simulink model "scenario_wind_integration"  (R2016b)
settings: Solver=ode23tb  StartTime=0.0  StopTime=2  RelTol=1e-3  EnableMultiTasking=on
undefined symbols (not defined in the file): sigbuilder_block
libraries: powerlib x28, powerlib_extras x7
settings Model: Creator=Amir  LastModifiedBy=Hosein
settings DataIOCC: LimitDataPoints=on  SaveFormat=Array  SignalLoggingSaveFormat=ModelDataLogs
settings OptimizationCC: ExpressionDepthLimit=2147483647  LifeSpan=inf
settings DebuggingCC: UnderspecifiedInitializationDetection=Classic  MergeDetectMultiDrivingBlocksExec=none  SolverPrmCheckMsg=warning  FcnCallInpInsideContextMsg=warning  StateNameClashWarn=warning  StrictBusMsg=Warning  SFUnexpectedBacktrackingDiag=warning  SFNoUnconditionalDefaultTransitionDiag=warning  SFExecutionAtInitializationDiag=none
settings HardwareCC: ProdBitPerPointer=32  ProdBitPerSizeT=32  ProdBitPerPtrDiffT=32  ProdLargestAtomicFloat=None  ProdIntDivRoundTo=Undefined  ProdEndianess=Unspecified  ProdWordSize=32  ProdHWDeviceType=32-bit Generic
settings ModelReferenceCC: PropagateSignalLabelsOutOfModel=off
settings GRTTargetCC: TargetLangStandard=C89/C90 (ANSI)  CombineOutputUpdateFcns=off  GRTInterface=on
settings ConfigComp: CovMetricSettings=dw  CovHtmlReporting=on  CovSaveCumulativeToWorkspaceVar=on  CovSaveSingleToWorkspaceVar=on  CovExternalEMLEnable=off

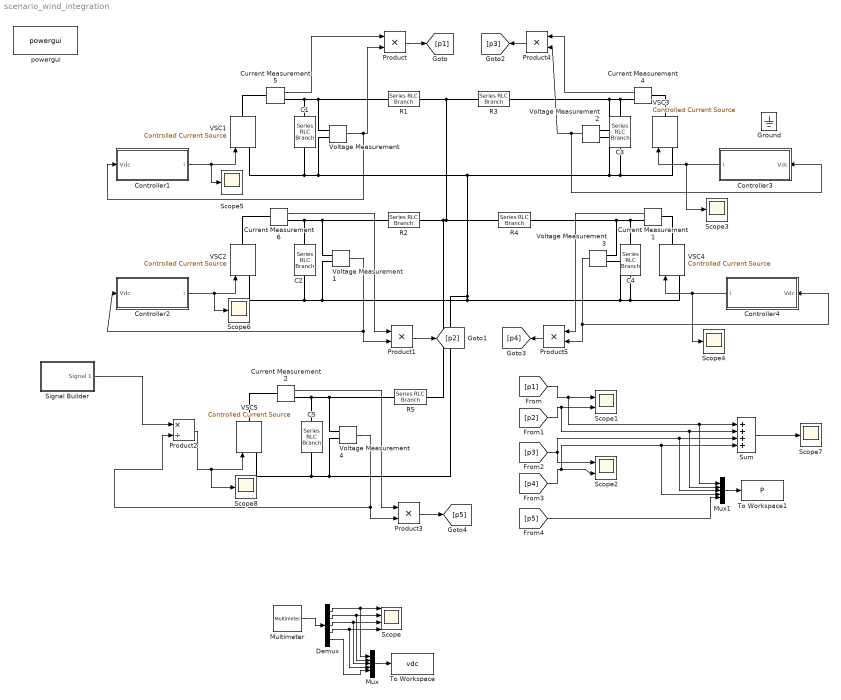
== system scenario_wind_integration ==
  C{1..5} (5 alike) : powerlib/Elements/Series RLC Branch  LConnTagsString=__new0  RConnTagsString=__new0  BranchType=C  Resistance=1  Inductance=1e-3  SetiL0=off  InitialCurrent=0  Capacitance=75e-6  Setx0=on  InitialVoltage=100e3  Measurements=Branch voltage
  Controller1 : Subsystem
  Controller2 : Subsystem
  Controller3 : Subsystem
  Controller4 : Subsystem
  Current Measurement{1..2,4..6} (5 alike) : powerlib/Measurements/Current Measurement  PhasorSimulation=off  OutputType=Complex  PSBequivalent=0
  Demux : Demux  Outputs=5
  Ground : powerlib/Elements/Ground  LConnTagsString=a
  Multimeter : powerlib/Measurements/Multimeter  PhasorSimulation=off  OutputType=Complex  sel=[1 2 3 4 5]  L=5  Gain=[1 1 1 1 1]  yselected={'Ub: C1','Ub: C2','Ub: C3','Ub: C4','Ub: C5'};  PSBOutputType=1  PSBequivalent=0  AxesSetting=[0,0.1,-100,100]  Display=0  SavedBlockNames=-11
  Mux : Mux  Inputs=5
  Mux1 : Mux  Inputs=5
  Product{,1,3..5} (5 alike) : Product  RndMeth=Zero
  Product2 : Product  Inputs=*/  RndMeth=Zero
  R1 : powerlib/Elements/Series RLC Branch  LConnTagsString=__new0  RConnTagsString=__new0  BranchType=R  Resistance=1.78  Inductance=141.5e-3  SetiL0=off  InitialCurrent=0  Capacitance=1e-6  Setx0=off  InitialVoltage=0  Measurements=None
  R2 : powerlib/Elements/Series RLC Branch  LConnTagsString=__new0  RConnTagsString=__new0  BranchType=R  Resistance=1.78  Inductance=141.5e-3  SetiL0=on  InitialCurrent=-1  Capacitance=1e-6  Setx0=off  InitialVoltage=0  Measurements=None
  R3 : powerlib/Elements/Series RLC Branch  LConnTagsString=__new0  RConnTagsString=__new0  BranchType=R  Resistance=1.78*0.5  Inductance=141.5e-3*0.5  SetiL0=on  InitialCurrent=0.5  Capacitance=1e-6  Setx0=off  InitialVoltage=0  Measurements=None
  R4 : powerlib/Elements/Series RLC Branch  LConnTagsString=__new0  RConnTagsString=__new0  BranchType=R  Resistance=1.78*0.75  Inductance=141.5e-3*0.75  SetiL0=on  InitialCurrent=0.5  Capacitance=1e-6  Setx0=off  InitialVoltage=0  Measurements=None
  R5 : powerlib/Elements/Series RLC Branch  LConnTagsString=__new0  RConnTagsString=__new0  BranchType=R  Resistance=1.78  Inductance=141.5e-3  SetiL0=on  InitialCurrent=-1  Capacitance=1e-6  Setx0=off  InitialVoltage=0  Measurements=None
  Scope : Scope  NumInputPorts=4
  Scope1 : Scope  NumInputPorts=2
  Scope2 : Scope  NumInputPorts=2
  Scope{3..8} (6 alike) : Scope
  Signal Builder : Subsystem  Tag=STV Subsys  LoadFcn=sigbuilder_block('load');  StartFcn=sigbuilder_block('start');  StopFcn=sigbuilder_block('stop');  ClipboardFcn=sigbuilder_block('clipboard');  mask(Sigbuilder block){tuvar=[0:10]}
      mask help: Sigbuilder GUI
      mask init:
      | if ~strcmp(get_param(bdroot(gcbh),'SimulationStatus'),'stopped') tuvar = sigbuilder_block('maskInit'); end
      settings: CopyFcn=sigbuilder_block('copy');  DeleteFcn=sigbuilder_block('delete');  ModelCloseFcn=sigbuilder_block('modelClose');  PreSaveFcn=sigbuilder_block('preSave');  PauseFcn=sigbuilder_block('pause')  ContinueFcn=sigbuilder_block('continue')  NameChangeFcn=sigbuilder_block('namechange');  OpenFcn=sigbuilder_block('open',[440.4 121.2 544.2 396 ]);  CloseFcn=sigbuilder_block('close');
      mask Display: plot(0,0,100,100,[10,10,40,40,10],[80,20,20,80,80],[40,10],[50,50], [40,27,10],[65,72,56],[40,25,25,10],[28,28,43,43]);
  Sum : Sum  Inputs=4
  To Workspace : ToWorkspace  VariableName=vdc  SampleTime=-1
  To Workspace1 : ToWorkspace  VariableName=P  SampleTime=-1
  VSC{1..5} (5 alike) : powerlib/Electrical Sources/Controlled Current Source  Initialize=on  Source_Type=AC  Amplitude=0  Phase=0  Frequency=0  Measurements=None
  Voltage Measurement{,1..4} (5 alike) : powerlib/Measurements/Voltage Measurement  PhasorSimulation=off  OutputType=Complex  PSBequivalent=0
  powergui : powerlib/powergui  Priority=1  SimulationMode=Discrete  SolverType=Tustin/Backward Euler (TBE)  SampleTime=1e-4  frequency=60  SPID=off  DisableSnubberDevices=off  DisableRonSwitches=off  DisableVfSwitches=off  SwTol=0  DisplayEquations=off  Interpol=off  ExternalGateDelay=off  methode=off  Ts=0  FunctionMessages=off  echomessages=off  HookPort=off  EnableUseOfTLC=off  x0status=blocks  frequencyindice=0  Pbase=100e6  ErrMax=1e-4  Iterations=50  UnitsV=kV  UnitsW=MW  buscounter=0  RestoreLinks=warning  ResistiveCurrentMeasurement=off  Frange=[0:2:500]  Ylog=off  Xlog=on  ShowGrid=off  save=off  variable=ZData  structure=0  ZoomFFT=on  StartTime=0.0  cycles=1  DisplayStyle=1  fundamental=60  FreqAxis=off  MaxFrequency=1000  frequencyindicesteady=1  RmsSteady=1  display=off
  wires:
  Controller4/1(i) -> VSC4/1, Scope4/1
  Controller3/1(i) -> VSC3/1, Scope3/1
  Controller1/1(i) -> VSC1/1, Scope5/1
  Controller2/1(i) -> VSC2/1, Scope6/1
  Multimeter/1 -> Demux/1
  Demux/1 -> Scope/1, Mux/1
  Demux/2 -> Scope/2, Mux/2
  Demux/3 -> Scope/3, Mux/3
  Demux/4 -> Scope/4, Mux/4
  Voltage Measurement/1 -> Product/2, Controller1/1(Vdc)
  Current Measurement6/1 -> Product1/1
  Voltage Measurement1/1 -> Product1/2, Controller2/1(Vdc)
  Product/1 -> [p1]
  Product1/1 -> [p2]
  [p1] -> Scope1/1, Sum/1, Mux1/1
  [p2] -> Scope1/2, Sum/2, Mux1/2
  Voltage Measurement2/1 -> Product4/2, Controller3/1(Vdc)
  Voltage Measurement3/1 -> Product5/2, Controller4/1(Vdc)
  Current Measurement4/1 -> Product4/1
  Current Measurement1/1 -> Product5/1
  Product4/1 -> [p3]
  Product5/1 -> [p4]
  [p3] -> Scope2/1, Sum/3, Mux1/3
  [p4] -> Scope2/2, Sum/4, Mux1/4
  Sum/1 -> Scope7/1
  Current Measurement5/1 -> Product/1
  Mux/1 -> To Workspace/1
  Signal Builder/1(Signal 1) -> Product2/1
  Mux1/1 -> To Workspace1/1
  Product2/1 -> VSC5/1, Scope8/1
  Current Measurement2/1 -> Product3/1
  Voltage Measurement4/1 -> Product3/2, Product2/2
  Product3/1 -> [p5]
  [p5] -> Mux1/5
  Demux/5 -> Mux/5
  connections:
  R1/LConn1 -- C1/LConn1 -- Current Measurement5/RConn1 -- Voltage Measurement/LConn1
  VSC1/LConn1 -- C1/RConn1 -- Voltage Measurement/LConn2 -- VSC3/LConn1 -- C3/RConn1 -- Voltage Measurement2/LConn2 -- VSC2/LConn1 -- C2/RConn1 -- Voltage Measurement1/LConn2 -- VSC4/LConn1 -- C4/RConn1 -- Voltage Measurement3/LConn2 -- Voltage Measurement4/LConn2 -- C5/RConn1 -- VSC5/LConn1
  R2/RConn1 -- R4/LConn1 -- R1/RConn1 -- R3/LConn1 -- R5/RConn1
  R3/RConn1 -- Voltage Measurement2/LConn1 -- C3/LConn1 -- Current Measurement4/RConn1
  R2/LConn1 -- C2/LConn1 -- Current Measurement6/RConn1 -- Voltage Measurement1/LConn1
  R4/RConn1 -- C4/LConn1 -- Current Measurement1/RConn1 -- Voltage Measurement3/LConn1
  Current Measurement5/LConn1 -- VSC1/RConn1
  Current Measurement6/LConn1 -- VSC2/RConn1
  Current Measurement1/LConn1 -- VSC4/RConn1
  Current Measurement4/LConn1 -- VSC3/RConn1
  R5/LConn1 -- Voltage Measurement4/LConn1 -- C5/LConn1 -- Current Measurement2/RConn1
  Current Measurement2/LConn1 -- VSC5/RConn1

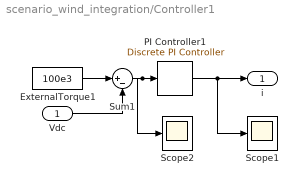
== system scenario_wind_integration/Controller1 ==
  Vdc : Inport
  ExternalTorque1 : Constant  Value=100e3
  PI Controller1 : powerlib_extras/Discrete  Control Blocks/Discrete PI Controller  Kp=10  Ki=10  Par_Limits=[0 -1000]  Init=0  Ts=1e-4
  Scope1 : Scope
  Scope2 : Scope
  Sum1 : Sum  Inputs=|+-
  i : Outport
  wires:
  ExternalTorque1/1 -> Sum1/1
  Vdc/1 -> Sum1/2
  Sum1/1 -> PI Controller1/1, Scope2/1
  PI Controller1/1 -> i/1, Scope1/1

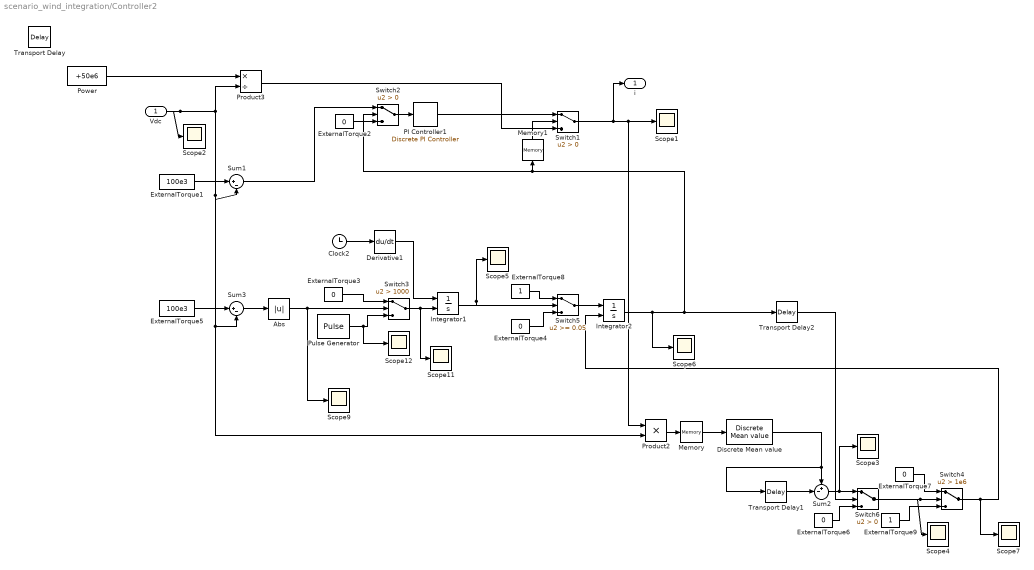
== system scenario_wind_integration/Controller2 ==
  Vdc : Inport
  Abs : Abs
  Clock2 : Clock
  Derivative1 : Derivative
  Discrete Mean value : powerlib_extras/Discrete Measurements/Discrete  Mean value  Freq=100  Vinit=0  Ts=1e-4
  ExternalTorque1 : Constant  Value=100e3
  ExternalTorque{2..4,6..7} (5 alike) : Constant  Value=0
  ExternalTorque5 : Constant  Value=100e3
  ExternalTorque8 : Constant
  ExternalTorque9 : Constant
  Integrator1 : Integrator  ExternalReset=either
  Integrator2 : Integrator  ExternalReset=either
  Memory : Memory
  Memory1 : Memory
  PI Controller1 : powerlib_extras/Discrete  Control Blocks/Discrete PI Controller  Kp=10  Ki=10  Par_Limits=[1000 -1000]  Init=0  Ts=1e-4
  Power : Constant  Value=+50e6
  Product2 : Product  Inputs=**  RndMeth=Zero
  Product3 : Product  Inputs=*/  RndMeth=Zero
  Pulse Generator : DiscretePulseGenerator  PulseType=Time based  Period=1e-4  PulseWidth=50
  Scope{1..7,9,11..12} (10 alike) : Scope
  Sum1 : Sum  Inputs=|+-
  Sum2 : Sum  Inputs=+-|
  Sum3 : Sum  Inputs=|+-
  Switch1 : Switch  Criteria=u2 > Threshold
  Switch2 : Switch  Criteria=u2 > Threshold
  Switch3 : Switch  Criteria=u2 > Threshold  Threshold=1000
  Switch4 : Switch  Criteria=u2 > Threshold  Threshold=1e6
  Switch5 : Switch  Threshold=0.05
  Switch6 : Switch  Criteria=u2 > Threshold
  Transport Delay : TransportDelay  DelayTime=0.05
  Transport Delay1 : TransportDelay  DelayTime=0.001
  Transport Delay2 : TransportDelay  DelayTime=0.1
  i : Outport
  wires:
  Sum1/1 -> Switch2/1
  ExternalTorque1/1 -> Sum1/1
  Power/1 -> Product3/1
  Product3/1 -> Switch1/3
  Switch2/1 -> PI Controller1/1
  PI Controller1/1 -> Switch1/1
  ExternalTorque2/1 -> Switch2/3
  Switch1/1 -> i/1, Scope1/1, Product2/1
  Switch3/1 -> Integrator1/2, Scope11/1
  Pulse Generator/1 -> Switch3/3, Scope12/1
  ExternalTorque3/1 -> Switch3/1
  Clock2/1 -> Derivative1/1
  Derivative1/1 -> Integrator1/1
  Abs/1 -> Switch3/2, Scope9/1
  Integrator1/1 -> Scope5/1, Switch5/2
  ExternalTorque4/1 -> Switch5/3
  Switch5/1 -> Integrator2/1
  ExternalTorque8/1 -> Switch5/1
  Integrator2/1 -> Scope6/1, Switch2/2, Memory1/1, Transport Delay2/1
  Vdc/1 -> Product3/2, Sum1/2, Product2/2, Sum3/2, Scope2/1
  Product2/1 -> Memory/1
  ExternalTorque9/1 -> Switch4/3
  ExternalTorque7/1 -> Switch4/1
  Discrete Mean value/1 -> Sum2/1, Transport Delay1/1
  Memory/1 -> Discrete Mean value/1
  Sum3/1 -> Abs/1
  ExternalTorque5/1 -> Sum3/1
  Memory1/1 -> Switch1/2
  Transport Delay1/1 -> Sum2/2
  Sum2/1 -> Switch6/1, Scope3/1
  Switch6/1 -> Switch4/2, Scope4/1
  ExternalTorque6/1 -> Switch6/3
  Switch4/1 -> Scope7/1, Integrator2/2
  Transport Delay2/1 -> Switch6/2

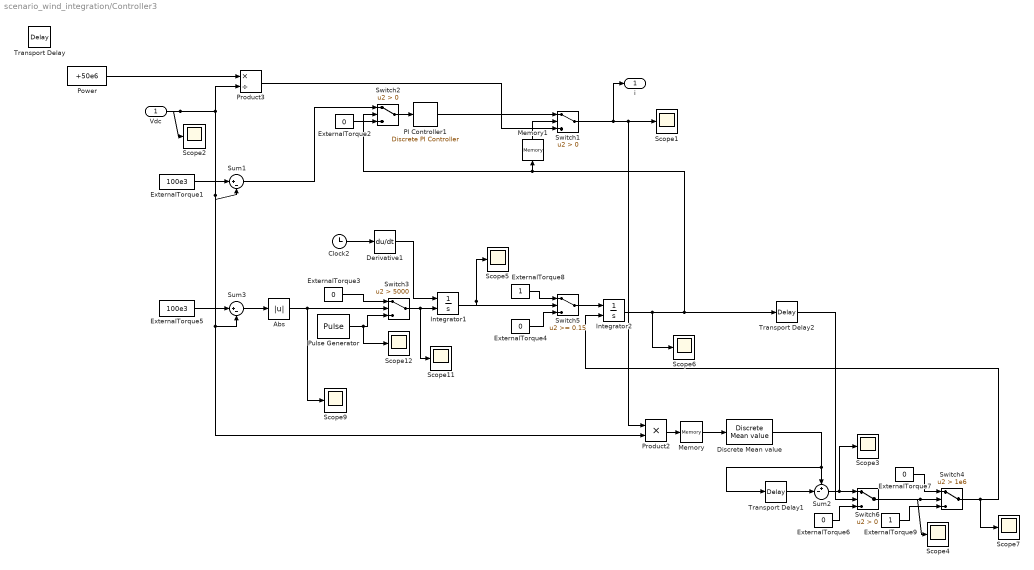
== system scenario_wind_integration/Controller3 ==
  Vdc : Inport
  Abs : Abs
  Clock2 : Clock
  Derivative1 : Derivative
  Discrete Mean value : powerlib_extras/Discrete Measurements/Discrete  Mean value  Freq=100  Vinit=0  Ts=1e-4
  ExternalTorque1 : Constant  Value=100e3
  ExternalTorque{2..4,6..7} (5 alike) : Constant  Value=0
  ExternalTorque5 : Constant  Value=100e3
  ExternalTorque8 : Constant
  ExternalTorque9 : Constant
  Integrator1 : Integrator  ExternalReset=either
  Integrator2 : Integrator  ExternalReset=either
  Memory : Memory
  Memory1 : Memory
  PI Controller1 : powerlib_extras/Discrete  Control Blocks/Discrete PI Controller  Kp=10  Ki=10  Par_Limits=[1000 -1000]  Init=0  Ts=1e-4
  Power : Constant  Value=+50e6
  Product2 : Product  Inputs=**  RndMeth=Zero
  Product3 : Product  Inputs=*/  RndMeth=Zero
  Pulse Generator : DiscretePulseGenerator  PulseType=Time based  Period=1e-4  PulseWidth=50
  Scope{1..7,9,11..12} (10 alike) : Scope
  Sum1 : Sum  Inputs=|+-
  Sum2 : Sum  Inputs=+-|
  Sum3 : Sum  Inputs=|+-
  Switch1 : Switch  Criteria=u2 > Threshold
  Switch2 : Switch  Criteria=u2 > Threshold
  Switch3 : Switch  Criteria=u2 > Threshold  Threshold=5000
  Switch4 : Switch  Criteria=u2 > Threshold  Threshold=1e6
  Switch5 : Switch  Threshold=0.15
  Switch6 : Switch  Criteria=u2 > Threshold
  Transport Delay : TransportDelay  DelayTime=0.05
  Transport Delay1 : TransportDelay  DelayTime=0.001
  Transport Delay2 : TransportDelay  DelayTime=0.1
  i : Outport
  wires:
  Transport Delay2/1 -> Switch6/2
  Switch4/1 -> Integrator2/2, Scope7/1
  ExternalTorque6/1 -> Switch6/3
  Switch6/1 -> Scope4/1, Switch4/2
  Sum2/1 -> Scope3/1, Switch6/1
  Transport Delay1/1 -> Sum2/2
  Memory1/1 -> Switch1/2
  ExternalTorque5/1 -> Sum3/1
  Sum3/1 -> Abs/1
  Memory/1 -> Discrete Mean value/1
  Discrete Mean value/1 -> Transport Delay1/1, Sum2/1
  ExternalTorque7/1 -> Switch4/1
  ExternalTorque9/1 -> Switch4/3
  Product2/1 -> Memory/1
  Vdc/1 -> Scope2/1, Sum3/2, Product2/2, Sum1/2, Product3/2
  Integrator2/1 -> Transport Delay2/1, Memory1/1, Switch2/2, Scope6/1
  ExternalTorque8/1 -> Switch5/1
  Switch5/1 -> Integrator2/1
  ExternalTorque4/1 -> Switch5/3
  Integrator1/1 -> Switch5/2, Scope5/1
  Abs/1 -> Scope9/1, Switch3/2
  Derivative1/1 -> Integrator1/1
  Clock2/1 -> Derivative1/1
  ExternalTorque3/1 -> Switch3/1
  Pulse Generator/1 -> Scope12/1, Switch3/3
  Switch3/1 -> Scope11/1, Integrator1/2
  Switch1/1 -> Product2/1, Scope1/1, i/1
  ExternalTorque2/1 -> Switch2/3
  PI Controller1/1 -> Switch1/1
  Switch2/1 -> PI Controller1/1
  Product3/1 -> Switch1/3
  Power/1 -> Product3/1
  ExternalTorque1/1 -> Sum1/1
  Sum1/1 -> Switch2/1

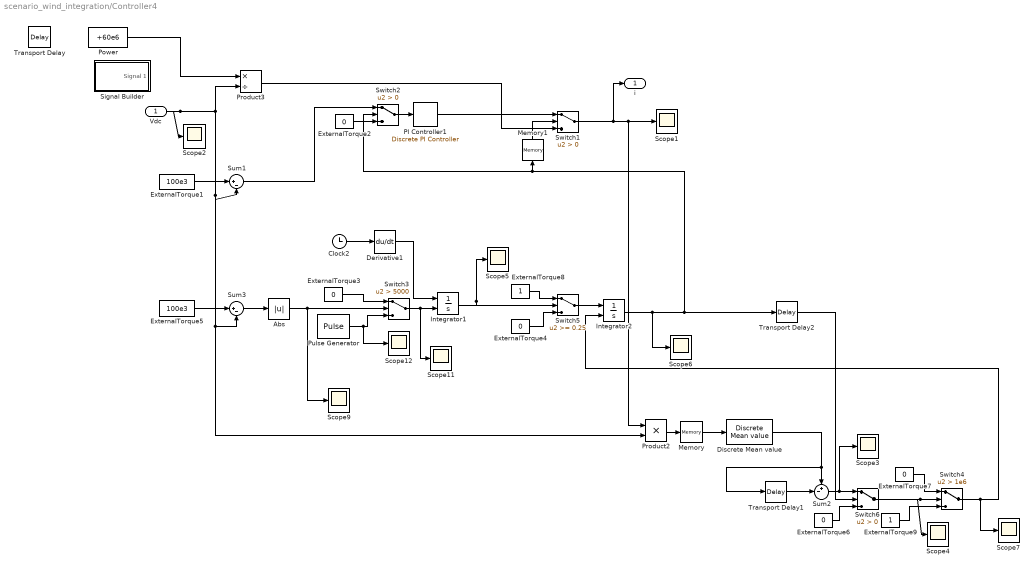
== system scenario_wind_integration/Controller4 ==
  Vdc : Inport
  Abs : Abs
  Clock2 : Clock
  Derivative1 : Derivative
  Discrete Mean value : powerlib_extras/Discrete Measurements/Discrete  Mean value  Freq=100  Vinit=0  Ts=1e-4
  ExternalTorque1 : Constant  Value=100e3
  ExternalTorque{2..4,6..7} (5 alike) : Constant  Value=0
  ExternalTorque5 : Constant  Value=100e3
  ExternalTorque8 : Constant
  ExternalTorque9 : Constant
  Integrator1 : Integrator  ExternalReset=either
  Integrator2 : Integrator  ExternalReset=either
  Memory : Memory
  Memory1 : Memory
  PI Controller1 : powerlib_extras/Discrete  Control Blocks/Discrete PI Controller  Kp=10  Ki=10  Par_Limits=[1000 -1000]  Init=0  Ts=1e-4
  Power : Constant  Value=+60e6
  Product2 : Product  Inputs=**  RndMeth=Zero
  Product3 : Product  Inputs=*/  RndMeth=Zero
  Pulse Generator : DiscretePulseGenerator  PulseType=Time based  Period=1e-4  PulseWidth=50
  Scope{1..7,9,11..12} (10 alike) : Scope
  Signal Builder : Subsystem  Tag=STV Subsys  LoadFcn=sigbuilder_block('load');  StartFcn=sigbuilder_block('start');  StopFcn=sigbuilder_block('stop');  ClipboardFcn=sigbuilder_block('clipboard');  mask(Sigbuilder block){tuvar=[0:10]}
      mask help: Sigbuilder GUI
      mask init:
      | if ~strcmp(get_param(bdroot(gcbh),'SimulationStatus'),'stopped') tuvar = sigbuilder_block('maskInit'); end
      settings: CopyFcn=sigbuilder_block('copy');  DeleteFcn=sigbuilder_block('delete');  ModelCloseFcn=sigbuilder_block('modelClose');  PreSaveFcn=sigbuilder_block('preSave');  PauseFcn=sigbuilder_block('pause')  ContinueFcn=sigbuilder_block('continue')  NameChangeFcn=sigbuilder_block('namechange');  OpenFcn=sigbuilder_block('open',[437.25 199.5 550.5 399.75 ]);  CloseFcn=sigbuilder_block('close');
      mask Display: plot(0,0,100,100,[10,10,40,40,10],[80,20,20,80,80],[40,10],[50,50], [40,27,10],[65,72,56],[40,25,25,10],[28,28,43,43]);
  Sum1 : Sum  Inputs=|+-
  Sum2 : Sum  Inputs=+-|
  Sum3 : Sum  Inputs=|+-
  Switch1 : Switch  Criteria=u2 > Threshold
  Switch2 : Switch  Criteria=u2 > Threshold
  Switch3 : Switch  Criteria=u2 > Threshold  Threshold=5000
  Switch4 : Switch  Criteria=u2 > Threshold  Threshold=1e6
  Switch5 : Switch  Threshold=0.25
  Switch6 : Switch  Criteria=u2 > Threshold
  Transport Delay : TransportDelay  DelayTime=0.05
  Transport Delay1 : TransportDelay  DelayTime=0.001
  Transport Delay2 : TransportDelay  DelayTime=0.1
  i : Outport
  wires:
  Sum1/1 -> Switch2/1
  ExternalTorque1/1 -> Sum1/1
  Product3/1 -> Switch1/3
  Switch2/1 -> PI Controller1/1
  PI Controller1/1 -> Switch1/1
  ExternalTorque2/1 -> Switch2/3
  Switch1/1 -> i/1, Scope1/1, Product2/1
  Switch3/1 -> Integrator1/2, Scope11/1
  Pulse Generator/1 -> Switch3/3, Scope12/1
  ExternalTorque3/1 -> Switch3/1
  Clock2/1 -> Derivative1/1
  Derivative1/1 -> Integrator1/1
  Abs/1 -> Switch3/2, Scope9/1
  Integrator1/1 -> Scope5/1, Switch5/2
  ExternalTorque4/1 -> Switch5/3
  Switch5/1 -> Integrator2/1
  ExternalTorque8/1 -> Switch5/1
  Integrator2/1 -> Scope6/1, Switch2/2, Memory1/1, Transport Delay2/1
  Vdc/1 -> Product3/2, Sum1/2, Product2/2, Sum3/2, Scope2/1
  Product2/1 -> Memory/1
  ExternalTorque9/1 -> Switch4/3
  ExternalTorque7/1 -> Switch4/1
  Discrete Mean value/1 -> Sum2/1, Transport Delay1/1
  Memory/1 -> Discrete Mean value/1
  Sum3/1 -> Abs/1
  ExternalTorque5/1 -> Sum3/1
  Memory1/1 -> Switch1/2
  Transport Delay1/1 -> Sum2/2
  Sum2/1 -> Switch6/1, Scope3/1
  Switch6/1 -> Switch4/2, Scope4/1
  ExternalTorque6/1 -> Switch6/3
  Switch4/1 -> Scope7/1, Integrator2/2
  Transport Delay2/1 -> Switch6/2
  Power/1 -> Product3/1

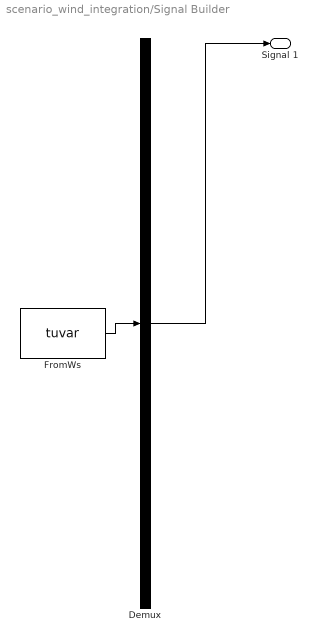
== system scenario_wind_integration/Signal Builder ==
  Demux : Demux  Tag=STV Demux  Outputs=1
  FromWs : FromWorkspace  Tag=STV FromWs  VariableName=tuvar  SampleTime=0
      SigBuilderData=|
      | common.afterFinalStr = 'Extrapolate'
      | common.sampleTime = 0
      | dataSet.timeRange = [0 2]
      | dataSet.name = 'Group 1'
      | sbobj.Groups.Name = 'Group 1'
      | sbobj.Groups.Signals.Name = 'Signal 1'
      | sbobj.Groups.Signals.XData = [0 0.405 0.405 1 1 2]
      | sbobj.Groups.Signals.YData = [20000 20000 30100 30100 9800 9800]
      | sbobj.Groups.TimeRange = [0 2]
  Signal 1 : Outport  Tag=STV Outport
  wires:
  Demux/1 -> Signal 1/1
  FromWs/1 -> Demux/1

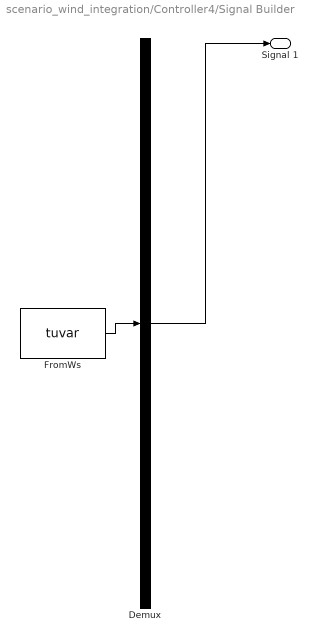
== system scenario_wind_integration/Controller4/Signal Builder ==
  Demux : Demux  Tag=STV Demux  Outputs=1
  FromWs : FromWorkspace  Tag=STV FromWs  VariableName=tuvar  SampleTime=0
      SigBuilderData=|
      | common.afterFinalStr = 'Extrapolate'
      | common.sampleTime = 0
      | dataSet.timeRange = [0 2]
      | dataSet.name = 'Group 1'
      | sbobj.Groups.Name = 'Group 1'
      | sbobj.Groups.Signals.Name = 'Signal 1'
      | sbobj.Groups.Signals.XData = [0 0.405 0.405 1 1 2]
      | sbobj.Groups.Signals.YData = [50000000 50000000 149000000 149000000 50000000 50000000]
  Signal 1 : Outport  Tag=STV Outport
  wires:
  Demux/1 -> Signal 1/1
  FromWs/1 -> Demux/1
